simulink model "modeloSimulink"  (R2018b)
settings: Solver=ode4  StartTime=0.0  StopTime=100  FixedStep=0.04  RelTol=1e-3
libraries: simulink x9, Controllers x1
settings Model: Creator=root  LastModifiedBy=root

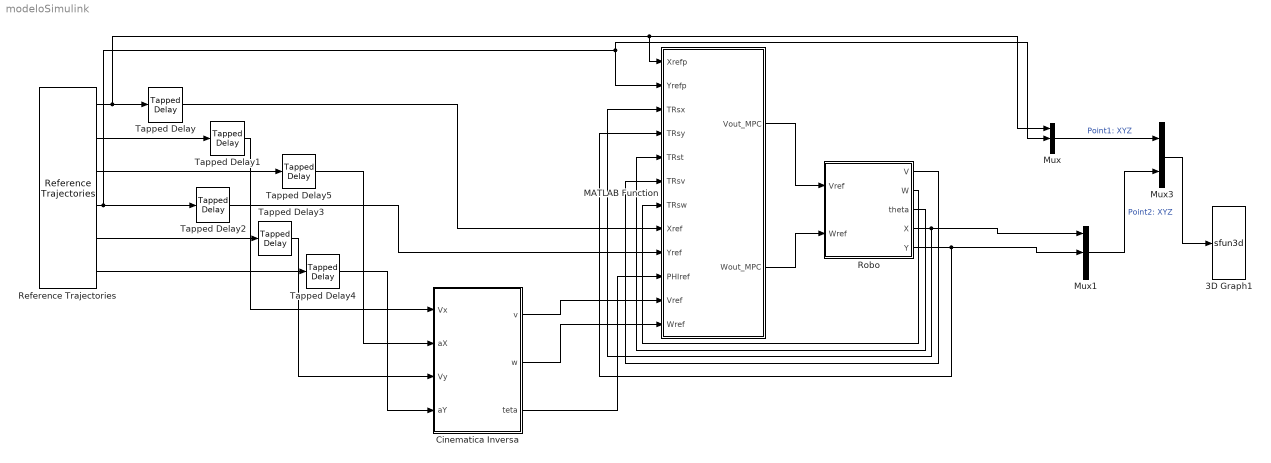
== system modeloSimulink ==
  3D Graph1 : S-Function  LoadFcn=if exist('sfun3d','file'), sfun3d([],[],[],'LoadBlock'); end  FunctionName=sfun3d  Parameters=ax,T,np,cp,gd,ls,mk,mx,hd,tb  SFunctionDeploymentMode=off  EnableBusSupport=off  mask(3D Graph){np=2, ax=[-4 4 -4 4 -3 3], mx=1e4, T=0.04, cp=[0 0 1], gd=on, hd=off, tb=off, ls=-, mk=none}
      mask prompts: np "Number of moving points (lines)"; ax "Range: [xmin xmax  ymin ymax zmin zmax]"; mx "Max number of points in each line"; T "Sampling Time"; cp "Camera position (use [0 0 1] for 2D XY view)"; gd "Grid (on|off)"; hd "HeadMarkers (on|off)"; tb "Toolbar (on|off)"; ls "LineStyle"; mk "LineMarker"
      mask help:
      | This block plots the position of several points in the XYZ space. The input contains the coordinates of all the points (x1,y1,z1,x2,y2,z2,...).
      | The number of moving points (lines), the XYZ ranges, sampling time, camera position, and grid (among other things) can be set as mask parameters.
      settings: CopyFcn=if exist('sfun3d','file'), sfun3d([],[],[],'CopyBlock'); end  DeleteFcn=if exist('sfun3d','file'), sfun3d([],[],[],'DeleteBlock'); end  NameChangeFcn=if exist('sfun3d','file'), sfun3d([],[],[],'NameChange'); end
      mask Help:
      | This block plots the position of several points in the XYZ space. The input contains the coordinates of all the points (x1,y1,z1,x2,y2,z2,...).
      | The number of moving points (lines), the XYZ ranges, sampling time, camera position, and grid (among other things) can be set as mask parameters.
      mask TypeOptions ls: - | -- | : | -. | none
      mask TypeOptions mk: none | . | + | o | * | x | square | diamond | v | ^ | > | < | pentagram | hexagram
      mask Display: plot([.05 .95 .95 .05 .05],[.45 .45 .95 .95 .45], 0.5+cos(0:0.1:2*pi)*0.3,0.7+sin(0:0.1:2*pi)*0.2)
  "Cinematica Inversa " : MATLAB Function  TreatAsAtomicUnit=on
  MATLAB Function : MATLAB Function  TreatAsAtomicUnit=on
  Mux : Mux  Inputs=3
  Mux1 : Mux  Inputs=3
  Mux3 : Mux  Inputs=2
  Reference Trajectories : Controllers/Reference Trajectories  trajectory_type=1  wf=0.10  raio_ref_1=1  delta_raio=0  t_delta_raio=60  xd=[1, -1.5]
  Robo : Subsystem
  Tapped Delay{,1..5} (6 alike) : simulink/Discrete/Tapped Delay  vinit=0.0  samptime=-1  NumDelays=1  DelayOrder=Oldest  includeCurrent=off
  wires:
  Robo/1(V) -> MATLAB Function/6(TRsv)
  Robo/2(W) -> MATLAB Function/7(TRsw)
  Robo/4(X) -> MATLAB Function/3(TRsx), Mux1/1
  Robo/5(Y) -> MATLAB Function/4(TRsy), Mux1/2
  MATLAB Function/2(Wout_MPC) -> Robo/2("Wref ")
  MATLAB Function/1(Vout_MPC) -> Robo/1("Vref ")
  Mux1/1 -> Mux3/2  "Point2: XYZ"
  Mux/1 -> Mux3/1  "Point1: XYZ"
  Reference Trajectories/1 -> Tapped Delay/1, MATLAB Function/1(Xrefp), Mux/1
  Reference Trajectories/4 -> Tapped Delay2/1, MATLAB Function/2(Yrefp), Mux/2
  Robo/3(theta) -> MATLAB Function/5(TRst)
  Reference Trajectories/2 -> Tapped Delay1/1
  Reference Trajectories/5 -> Tapped Delay3/1
  Reference Trajectories/6 -> Tapped Delay4/1
  Reference Trajectories/3 -> Tapped Delay5/1
  Tapped Delay/1 -> MATLAB Function/8(Xref)
  Tapped Delay2/1 -> MATLAB Function/9(Yref)
  "Cinematica Inversa "/1(v) -> MATLAB Function/11(Vref)
  "Cinematica Inversa "/3(teta) -> MATLAB Function/10(PHIref)
  "Cinematica Inversa "/2(w) -> MATLAB Function/12(Wref)
  Tapped Delay4/1 -> "Cinematica Inversa "/4(aY)
  Tapped Delay3/1 -> "Cinematica Inversa "/3(Vy)
  Tapped Delay5/1 -> "Cinematica Inversa "/2(aX)
  Tapped Delay1/1 -> "Cinematica Inversa "/1(Vx)
  Mux3/1 -> 3D Graph1/1

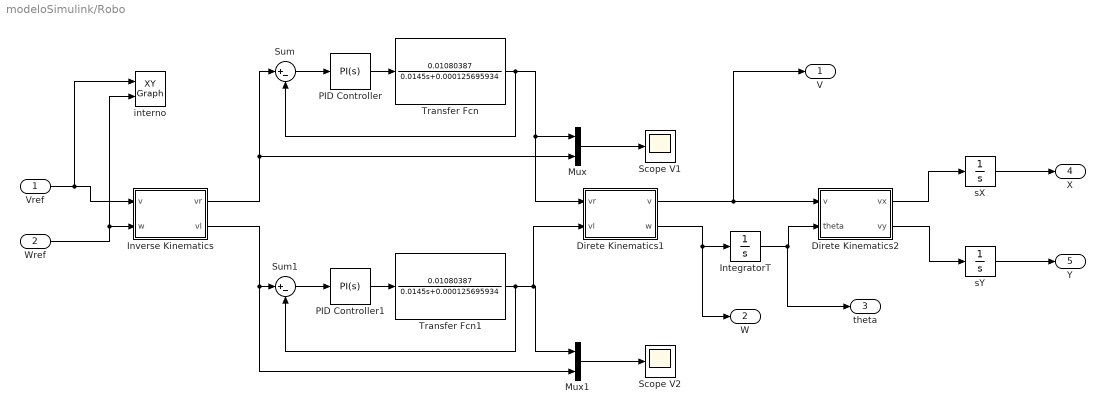
== system modeloSimulink/Robo ==
  "Vref " : Inport
  "Wref " : Inport  Port=2
  Direte Kinematics1 : MATLAB Function  TreatAsAtomicUnit=on
  Direte Kinematics2 : MATLAB Function  TreatAsAtomicUnit=on
  IntegratorT : Integrator
  Inverse Kinematics : MATLAB Function  TreatAsAtomicUnit=on
  Mux : Mux  Inputs=2
  Mux1 : Mux  Inputs=2
  PID Controller : simulink/Continuous/PID Controller  Controller=PI  Form=Parallel  TimeDomain=Continuous-time  SampleTime=-1  IntegratorMethod=Forward Euler  FilterMethod=Forward Euler  ControllerParametersSource=internal  P=0.8  I=0.06  D=0  UseFilter=on  N=100  TunerSelectOption=Transfer Function Based (PID Tuner App)  InitialConditionSource=internal  InitialConditionForIntegrator=0  InitialConditionForFilter=0  DifferentiatorICPrevScaledInput=0  ExternalReset=none  TrackingMode=off  Kt=1  LimitOutput=off  UpperSaturationLimit=inf  LowerSaturationLimit=-inf  LinearizeAsGain=on  AntiWindupMode=none  Kb=1  POutMin=[]  POutMax=[]  IOutMin=[]  IOutMax=[]  DOutMin=[]  DOutMax=[]  NOutMin=[]  NOutMax=[]  SumOutMin=[]  SumOutMax=[]  SaturationOutMin=[]  SaturationOutMax=[]  PParamMin=[]  PParamMax=[]  IParamMin=[]  IParamMax=[]  DParamMin=[]  DParamMax=[]  NParamMin=[]  NParamMax=[]  KbParamMin=[]  KbParamMax=[]  KtParamMin=[]  KtParamMax=[]  KbOutMin=[]  KbOutMax=[]  KtOutMin=[]  KtOutMax=[]  IntegratorOutMin=[]  IntegratorOutMax=[]  FilterOutMin=[]  FilterOutMax=[]  SumI1OutMin=[]  SumI1OutMax=[]  SumI2OutMin=[]  SumI2OutMax=[]  SumI3OutMin=[]  SumI3OutMax=[]  SumI4OutMin=[]  SumI4OutMax=[]  SumDOutMin=[]  SumDOutMax=[]  DifferentiatorOutMin=[]  DifferentiatorOutMax=[]  FilterDiffOutCoefMin=[]  FilterDiffOutCoefMax=[]  ReciprocalOutMin=[]  ReciprocalOutMax=[]  SumDenOutMin=[]  SumDenOutMax=[]  SumNumOutMin=[]  SumNumOutMax=[]  DivideOutMin=[]  DivideOutMax=[]  IntegratorContinuousStateAttributes=''  IntegratorStateMustResolveToSignalObject=off  IntegratorRTWStateStorageClass=Auto  FilterContinuousStateAttributes=''  FilterStateMustResolveToSignalObject=off  FilterRTWStateStorageClass=Auto  ParallelPVariant=InternalParameters  IdealPVariant=Disabled  IVariant=InternalParameters  DVariant=Disabled  IntegratorVariant=Continuous  SatVariant=Disabled  AWVariant=Passthrough  PCopyVariant=Disabled  TRVariant=Disabled  FdbkBlocksVariant=Forward  IdealPFdbkVariant=Disabled  SatFdbkVariant=Disabled  DerivativeFilterVariant=Disabled  NVariant=Disabled  NCopyVariant=Disabled_SignalSpec  FilterICVariant=Disabled  IntegratorICVariant=InternalICs  ExternalResetVariant=Disabled  TRSumVariant=Passthrough  SumFdbkVariant=Disabled  SumVariant=Sum_PI
  PID Controller1 : simulink/Continuous/PID Controller  Controller=PI  Form=Parallel  TimeDomain=Continuous-time  SampleTime=-1  IntegratorMethod=Forward Euler  FilterMethod=Forward Euler  ControllerParametersSource=internal  P=0.8  I=0.06  D=0  UseFilter=on  N=100  TunerSelectOption=Transfer Function Based (PID Tuner App)  InitialConditionSource=internal  InitialConditionForIntegrator=0  InitialConditionForFilter=0  DifferentiatorICPrevScaledInput=0  ExternalReset=none  TrackingMode=off  Kt=1  LimitOutput=off  UpperSaturationLimit=inf  LowerSaturationLimit=-inf  LinearizeAsGain=on  AntiWindupMode=none  Kb=1  POutMin=[]  POutMax=[]  IOutMin=[]  IOutMax=[]  DOutMin=[]  DOutMax=[]  NOutMin=[]  NOutMax=[]  SumOutMin=[]  SumOutMax=[]  SaturationOutMin=[]  SaturationOutMax=[]  PParamMin=[]  PParamMax=[]  IParamMin=[]  IParamMax=[]  DParamMin=[]  DParamMax=[]  NParamMin=[]  NParamMax=[]  KbParamMin=[]  KbParamMax=[]  KtParamMin=[]  KtParamMax=[]  KbOutMin=[]  KbOutMax=[]  KtOutMin=[]  KtOutMax=[]  IntegratorOutMin=[]  IntegratorOutMax=[]  FilterOutMin=[]  FilterOutMax=[]  SumI1OutMin=[]  SumI1OutMax=[]  SumI2OutMin=[]  SumI2OutMax=[]  SumI3OutMin=[]  SumI3OutMax=[]  SumI4OutMin=[]  SumI4OutMax=[]  SumDOutMin=[]  SumDOutMax=[]  DifferentiatorOutMin=[]  DifferentiatorOutMax=[]  FilterDiffOutCoefMin=[]  FilterDiffOutCoefMax=[]  ReciprocalOutMin=[]  ReciprocalOutMax=[]  SumDenOutMin=[]  SumDenOutMax=[]  SumNumOutMin=[]  SumNumOutMax=[]  DivideOutMin=[]  DivideOutMax=[]  IntegratorContinuousStateAttributes=''  IntegratorStateMustResolveToSignalObject=off  IntegratorRTWStateStorageClass=Auto  FilterContinuousStateAttributes=''  FilterStateMustResolveToSignalObject=off  FilterRTWStateStorageClass=Auto  ParallelPVariant=InternalParameters  IdealPVariant=Disabled  IVariant=InternalParameters  DVariant=Disabled  IntegratorVariant=Continuous  SatVariant=Disabled  AWVariant=Passthrough  PCopyVariant=Disabled  TRVariant=Disabled  FdbkBlocksVariant=Forward  IdealPFdbkVariant=Disabled  SatFdbkVariant=Disabled  DerivativeFilterVariant=Disabled  NVariant=Disabled  NCopyVariant=Disabled_SignalSpec  FilterICVariant=Disabled  IntegratorICVariant=InternalICs  ExternalResetVariant=Disabled  TRSumVariant=Passthrough  SumFdbkVariant=Disabled  SumVariant=Sum_PI
  Scope V1 : Scope
  Scope V2 : Scope
  Sum : Sum  Inputs=|+-
  Sum1 : Sum  Inputs=|+-
  Transfer Fcn : TransferFcn  Numerator=[0.01080387]  Denominator=[0.0145 0.000125695934]
  Transfer Fcn1 : TransferFcn  Numerator=[0.01080387]  Denominator=[0.0145 0.000125695934]
  interno : simulink/Sinks/XY Graph  xmin=-1  xmax=1  ymin=-1  ymax=1  st=-1
  sX : Integrator
  sY : Integrator
  V : Outport
  W : Outport  Port=2
  theta : Outport  Port=3
  X : Outport  Port=4
  Y : Outport  Port=5
  wires:
  Sum/1 -> PID Controller/1
  PID Controller/1 -> Transfer Fcn/1
  Transfer Fcn/1 -> Direte Kinematics1/1(vr), Mux/1, Sum/2
  Inverse Kinematics/1(vr) -> Sum/1, Mux/2
  Mux/1 -> Scope V1/1
  Mux1/1 -> Scope V2/1
  PID Controller1/1 -> Transfer Fcn1/1
  Sum1/1 -> PID Controller1/1
  Transfer Fcn1/1 -> Direte Kinematics1/2(vl), Mux1/1, Sum1/2
  Inverse Kinematics/2(vl) -> Mux1/2, Sum1/1
  Direte Kinematics1/1(v) -> Direte Kinematics2/1(v), V/1
  Direte Kinematics1/2(w) -> W/1, IntegratorT/1
  IntegratorT/1 -> theta/1, Direte Kinematics2/2(theta)
  Direte Kinematics2/2(vy) -> sY/1
  Direte Kinematics2/1(vx) -> sX/1
  sX/1 -> X/1
  sY/1 -> Y/1
  "Vref "/1 -> interno/1, Inverse Kinematics/1(v)
  "Wref "/1 -> interno/2, Inverse Kinematics/2(w)

== matlab function modeloSimulink/Robo/Direte Kinematics1 ==
  data: vr input; v output; vl input; w output
%function y = fcn(u)
function [v,w] = fcn(vr,vl)
    L = 2 * 0.17;
    v = (vr + vl)/2;
    w = (vr - vl)/L;
end

== matlab function modeloSimulink/Robo/Inverse Kinematics ==
  data: v input; vr output; w input; vl output
%function y = fcn(u)
function [vr,vl] = fcn(v,w)
    L = 2 * 0.17;
    vr = v + (w * L)/2;
    vl = v - (w * L)/2;
end

== matlab function modeloSimulink/Robo/Direte Kinematics2 ==
  data: v input; vx output; theta input; vy output
%function y = fcn(u)
function [vx,vy] = fcn(v,theta)
    vx = v * cos(theta);
    vy = v * sin(theta);
end

== matlab function modeloSimulink/MATLAB Function ==
  data: Xrefp input; Vout_MPC output; Yrefp input; TRsx input; TRsy input; TRst input; TRsv input; TRsw input; Xref input; Yref input; PHIref input; Vref input; Wref input; Wout_MPC output
function [Vout_MPC, Wout_MPC] = MPC(Xrefp, Yrefp, TRsx, TRsy, TRst, TRsv, TRsw,Xref, Yref, PHIref, Vref, Wref)
    % Parâmetros do controlador
    Vmax = 0.4;
    d = 0.23;
    N1 = 1;
    N2 = 10; %Horizonte de predição
    Nu = 2;  %Horizonte de controle
    L1 = 1;
    L2 = 2.5;
    L3 = 1;
    eta = 0.1;
    Imax = 15;
    I = 0;
    Delta = 0.1;
    
    % Parâmetros do Otimizador
    alpha = 0.015;
    
    % Vetores do Otimizador
    
    Jgrad      = zeros([4 1]);
    Jgrad_prev = zeros([4 1]);
    Jsteps     = zeros([8 1]);
    % Definição das variáveis de controle
    
    Ubest = zeros([2 2]);
    Uref  = zeros([2 2]);
    Uaux  = zeros([2 2]);
    
    % Criação de um struct para guardar o valor da iteração anterior do
    % controlador
    SimRob = struct('x',0,'y',0,'teta',0,'v',0,'w',0);
    
    % Inicialização das variáveis de controle
    
    %Saida de controle desejada
    Uref = [Vref Vref; Wref Wref];
    
    % Cálculo da trajetoria de referencia
    lTi = 0;
    
    [tPX,tPY,tPTeta] = calcRefTraj(lTi,TRsx,TRsy,TRst,Xref,Yref,PHIref,Vref,Wref,N2,Xrefp,Yrefp);
    
    % Atualiza o modelo do preditor
    SimRob.x = TRsx;
    SimRob.y = TRsy;
    SimRob.teta = TRst;
    SimRob.v = TRsv;
    SimRob.w = TRsw;
    
    % Loop de controle
    
    % Reliza a saturaçao da velocidade das rodas com base na velocidade
    % máxima
    Uref = scaleForSaturation(Uref,d,Nu,Vmax);
    
    Jatual = COST_FUNCTION(SimRob.x,SimRob.y,SimRob.teta,SimRob.v,SimRob.w,Uref,tPX,tPY,tPTeta,N1,N2,Nu,L1,L2,L3);
    Jbest = Jatual;    

   %Loop de otimização do Ubest que minimiza o Jbest
   while (I < Imax) && (Jatual > eta)
       Usteps = calcUsteps(Uref,Nu, Delta);
        for k = 0:1:Nu-1
            for j=1:1:4
                %Atribui velocidade para cada passo U
                for m = 0:1:Nu-1
                    if m == k
                        Uaux(1,m+1)= Usteps(1,(j+4*k));
                        Uaux(2,m+1)= Usteps(2,(j+4*k));
                    else
                        Uaux(1,m+1)=Uref(1,1);
                        Uaux(2,m+1)=Uref(2,1);
                    end 
                    
                end
                SimRob.x=TRsx;
                SimRob.y=TRsy;
                SimRob.teta=TRst;
                SimRob.v=TRsv;
                SimRob.w=TRsw;

                Uaux=scaleForSaturation(Uaux,d,Nu,Vmax);

                J = COST_FUNCTION(SimRob.x,SimRob.y,SimRob.teta,SimRob.v,SimRob.w,Uaux,tPX,tPY,tPTeta,N1,N2,Nu,L1,L2,L3);
                Jsteps(j+ 4*k,1) = J;
            
            end
        end
        
        % calculo do gradiente de J baseado no Jsteps
        for h=0:1:Nu-1
            Jgrad_prev(2*h+1,1) = Jgrad(2*h+1,1);
            Jgrad(2*h+1,1) = Jsteps(4*h+1,1)- Jsteps(4*h+2,1);
            Jgrad_prev(2*h+2,1) = Jgrad(2*h+2,1);
            Jgrad(2*h+2,1)=Jsteps(4*h+3,1)-Jsteps(4*h+4,1);
        end
    
        %Gradiente conjugado Algoritmo de Polak-Bibieri

        di=[0 0];
        x1=di;

        for z=0:1:Nu-1
            di(1)=Jgrad(2*z+1,1);
            di(2)=Jgrad(2*z+2,1);
            
            x1(1)=(Uref(1,z+1) - alpha*di(1));
            x1(2)=(Uref(2,z+1) - alpha*di(2));
            
            Jgrad_prev(2*z+1,1)=Jgrad(2*z+1,1);
            Jgrad(2*z+1,1)=Jsteps(4*z+1,1)-Jsteps(4*z+2,1);
            
            Jgrad_prev(2*z+2,1)=Jgrad(2*z+2,1);
            Jgrad(2*z+2,1)=Jsteps(4*z+3,1)-Jsteps(4*z+4,1);
            
            beta=0;
            
            if ((Jgrad(2*z+1,1)>=eta)||(Jgrad(2*z+2,1)>=eta))
                
                t1=(Jgrad(2*z+1,1)-Jgrad_prev(2*z+1,1));
                t2=(Jgrad(2*z+2,1)-Jgrad_prev(2*z+2,1));
                
                a1=(Jgrad(2*z+1,1)*t1);
                a2=(Jgrad(2*z+2,1)*t2);
               
                b1=(Jgrad_prev(2*z+1,1)*Jgrad_prev(2*z+1,1));
                b2=(Jgrad_prev(2*z+2,1)*Jgrad_prev(2*z+2,1));
                
                beta=((a1+a2)/(b1+b2));
            
            end
            
            Uref(1,z+1)=x1(1)+alpha*(-Jgrad(2*z+1,1)+beta*Jgrad_prev(2*z+1,1));

            Uref(2,z+1)=x1(2)+alpha*(-Jgrad(2*z+2,1)+beta*Jgrad_prev(2*z+2,1));
        end
        
        
        SimRob.x=TRsx;
        SimRob.y=TRsy;
        SimRob.teta=TRst;
        SimRob.v=TRsv;
        SimRob.w=TRsw;
        
        % ix SATURA A VELOCIDADE DAS RODAS QUE SERÃO USADAS NO PRÓXIMO LOOP
        % DE CONTROLE (while)
        
        Uref = scaleForSaturation(Uref,d,Nu,Vmax);
        
        Jatual = COST_FUNCTION(SimRob.x,SimRob.y,SimRob.teta,SimRob.v,SimRob.w,Uref,tPX,tPY,tPTeta,N1,N2,Nu,L1,L2,L3);
        
        if Jatual < Jbest
            Jbest = Jatual;
            Ubest = Uref;
        end
        I=I+1;
    end %END_WHILE      
    Vout_MPC = Ubest(1,1);
    Wout_MPC = Ubest(2,1);

== matlab function modeloSimulink/Cinematica Inversa  ==
  data: Vx input; v output; aX input; Vy input; aY input; w output; teta output
function [v,w,teta] = fnc(Vx, aX, Vy, aY)
  
    teta = atan2(Vy,Vx);
    
    v = sqrt(Vx^2 + Vy^2);
    
    w = (Vx*aY - Vy*aX)/(Vx^2 + Vy^2);

end
